simulink model "Copy_of_completemodel"  (R2020b)
settings: Solver=VariableStepAuto  StartTime=0.0  StopTime=170.0  RelTol=1e-3
values from neighbouring files (symbols this model uses):
  A = [-0.322 0.052 0.028 -1.12 0.002 ... (first row only)    [Problem2.m]
  B = [0 0 0 0 7.5]'    [Problem2.m]
  C = [1 0 0 0 0 ... (first row only)    [Problem2.m]
  k_dphi = (2*zeta_phi*omega_nphi-a_phi1)/a_phi2    [Problem2.m]
  k_ichi = (omega_nchi^2*V_g)/g    [Problem2.m]
  k_iphi = -0.6    [Problem2.m]
  k_pchi = (2*zeta_chi*omega_nchi*V_g)/g    [Problem2.m]
  k_pphi = -2    [Problem2.m]
settings Model: Creator=ingridnorland  LastModifiedBy=ingridnorland

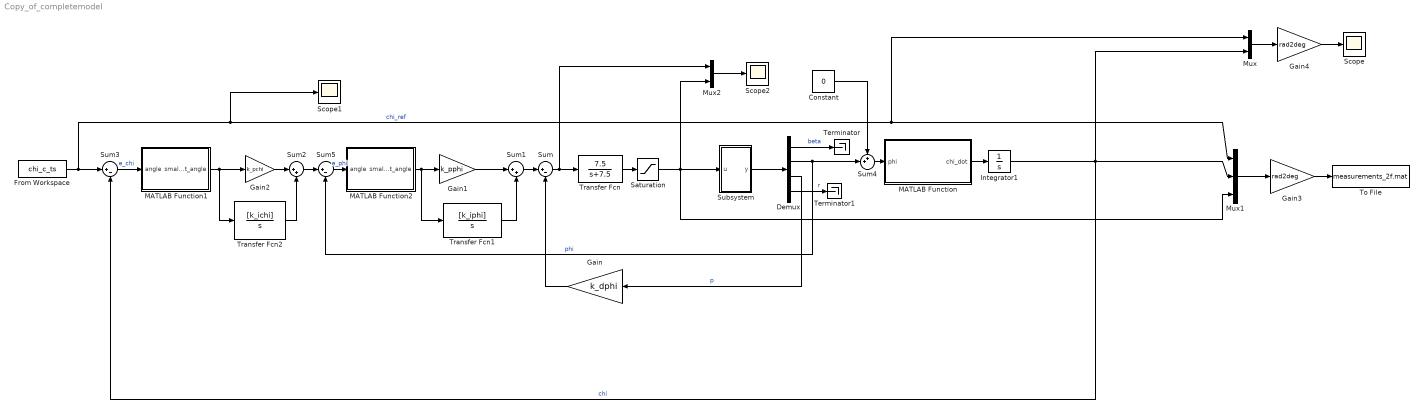
== system Copy_of_completemodel ==
  Constant : Constant  Value=0
  Demux : Demux
  From Workspace : FromWorkspace  VariableName=chi_c_ts
  Gain : Gain  Gain=k_dphi
  Gain1 : Gain  Gain=k_pphi
  Gain2 : Gain  Gain=k_pchi
  Gain3 : Gain  Gain=rad2deg
  Gain4 : Gain  Gain=rad2deg
  Integrator1 : Integrator
  MATLAB Function : MATLAB Function  TreatAsAtomicUnit=on
  MATLAB Function1 : MATLAB Function  TreatAsAtomicUnit=on
  MATLAB Function2 : MATLAB Function  TreatAsAtomicUnit=on
  Mux : Mux  Inputs=2
  Mux1 : Mux  Inputs=3
  Mux2 : Mux  Inputs=2
  Saturation : Saturate  UpperLimit=30*deg2rad  LowerLimit=-30*deg2rad
  Scope : Scope
  Scope1 : Scope
  Scope2 : Scope
  Subsystem : Subsystem
  Sum : Sum  Inputs=|+-
  Sum1 : Sum  Inputs=|++
  Sum2 : Sum  Inputs=|++
  Sum3 : Sum  Inputs=|+-
  Sum4 : Sum  Inputs=++|
  Sum5 : Sum  Inputs=|+-
  Terminator : Terminator
  Terminator1 : Terminator
  To File : ToFile  Filename=measurements_2f.mat  MatrixName=measurements
  Transfer Fcn : TransferFcn  Numerator=[7.5]  Denominator=[1 7.5]
  Transfer Fcn1 : TransferFcn  Numerator=[k_iphi]  Denominator=[1 0]
  Transfer Fcn2 : TransferFcn  Numerator=[k_ichi]  Denominator=[1 0]
  wires:
  Transfer Fcn2/1 -> Sum2/2
  Subsystem/1(y) -> Demux/1
  Gain/1 -> Sum/2
  Sum1/1 -> Sum/1
  Gain1/1 -> Sum1/1
  Transfer Fcn1/1 -> Sum1/2
  Sum/1 -> Transfer Fcn/1, Mux2/1
  Sum4/1 -> MATLAB Function/1(phi)
  Gain2/1 -> Sum2/1
  From Workspace/1 -> Sum3/1, Mux1/1, Mux/1, Scope1/1  "chi_ref"
  Sum2/1 -> Sum5/1
  Integrator1/1 -> Sum3/2, Mux1/2, Mux/2  "chi"
  Demux/2 -> Sum4/2, Sum5/2  "phi"
  Demux/3 -> Gain/1  "p"
  MATLAB Function/1(chi_dot) -> Integrator1/1
  Constant/1 -> Sum4/1
  Mux1/1 -> Gain3/1
  Gain3/1 -> To File/1
  Gain4/1 -> Scope/1
  Mux/1 -> Gain4/1
  Demux/1 -> Terminator/1  "beta"
  Mux2/1 -> Scope2/1
  Transfer Fcn/1 -> Saturation/1
  Saturation/1 -> Subsystem/1(u), Mux1/3, Mux2/2
  Sum5/1 -> MATLAB Function2/1(angle)  "e_phi"
  MATLAB Function2/1(smallest_angle) -> Transfer Fcn1/1, Gain1/1
  MATLAB Function1/1(smallest_angle) -> Gain2/1, Transfer Fcn2/1
  Sum3/1 -> MATLAB Function1/1(angle)  "e_chi"
  Demux/4 -> Terminator1/1  "r"

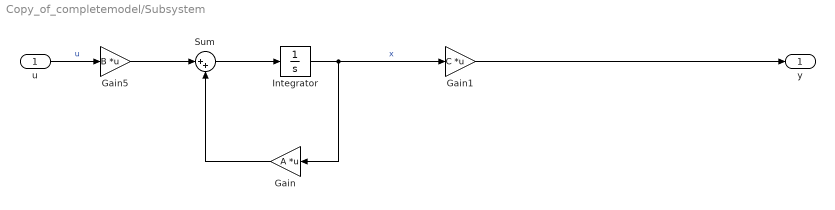
== system Copy_of_completemodel/Subsystem ==
  u : Inport
  Gain : Gain  Gain=A  Multiplication=Matrix(K*u)
  Gain1 : Gain  Gain=C  Multiplication=Matrix(K*u)
  Gain5 : Gain  Gain=B  Multiplication=Matrix(K*u)
  Integrator : Integrator
  Sum : Sum  Inputs=|++
  y : Outport
  wires:
  u/1 -> Gain5/1  "u"
  Gain5/1 -> Sum/1
  Sum/1 -> Integrator/1
  Integrator/1 -> Gain1/1, Gain/1  "x"
  Gain/1 -> Sum/2
  Gain1/1 -> y/1

== matlab function Copy_of_completemodel/MATLAB Function ==
  data: chi_dot output; phi input
function chi_dot = bank_to_turn(phi)
g= 9.81;
V_g = 580;
chi_dot = (g/V_g)*tan(phi);
end

== matlab function Copy_of_completemodel/MATLAB Function2 ==
  data: angle input; smallest_angle output
function smallest_angle = my_ssa(angle)

smallest_angle = ssa(angle,'rad');

== matlab function Copy_of_completemodel/MATLAB Function1 ==
  data: angle input; smallest_angle output
function smallest_angle = my_ssa(angle)

smallest_angle = ssa(angle,'rad');
